simulink model "linear_equation"  (R2025b)
settings: Solver=VariableStepAuto  StartTime=0.0  StopTime=10.0  RelTol=1e-3
undefined symbols (not defined in the file or in its folder): x, x1, x2, x3
settings Model: Creator=night  LastModifiedBy=night

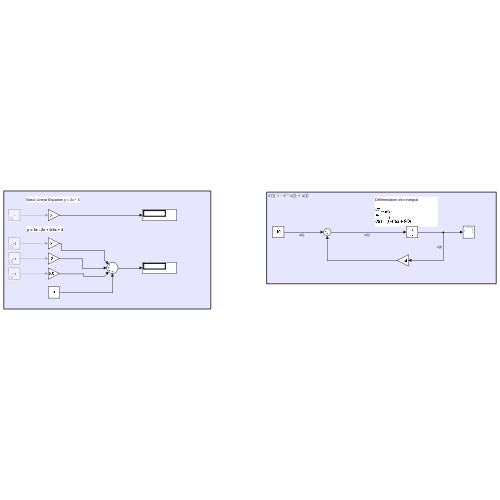
[thumbnail: Simulink's stored preview of the top-level diagram]
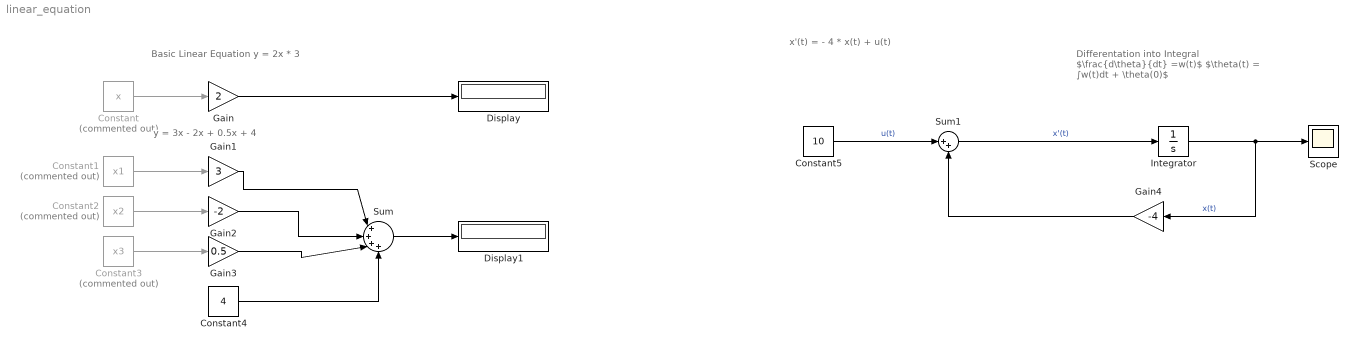
== system linear_equation ==
  note: Differentation into Integral
      |
      | $\frac{d\theta}{dt} =w(t)$
      | $\theta(t) = ∫w(t)dt + \theta(0)$
  note: x'(t) = - 4 * x(t) + u(t)
  note: y = 3x - 2x + 0.5x + 4
  note: Basic Linear Equation y = 2x * 3
  Constant : Constant  Commented=on  Value=x
  Constant1 : Constant  Commented=on  Value=x1
  Constant2 : Constant  Commented=on  Value=x2
  Constant3 : Constant  Commented=on  Value=x3
  Constant4 : Constant  Value=4
  Constant5 : Constant  Value=10
  Display : Display
  Display1 : Display
  Gain : Gain  Gain=2
  Gain1 : Gain  Gain=3
  Gain2 : Gain  Gain=-2
  Gain3 : Gain  Gain=0.5
  Gain4 : Gain  Gain=-4
  Integrator : Integrator
  Scope : Scope
      settings: ActiveDisplayYMinimum=-0.31249999999999989  ActiveDisplayYMaximum=2.8124999999999996
  Sum : Sum  Inputs=|++++
  Sum1 : Sum  Inputs=|++
  wires:
  Constant/1 -> Gain/1
  Gain/1 -> Display/1
  Gain1/1 -> Sum/1
  Constant1/1 -> Gain1/1
  Gain2/1 -> Sum/2
  Constant2/1 -> Gain2/1
  Gain3/1 -> Sum/3
  Constant3/1 -> Gain3/1
  Constant4/1 -> Sum/4
  Sum/1 -> Display1/1
  Constant5/1 -> Sum1/1  "u(t)"
  Gain4/1 -> Sum1/2
  Sum1/1 -> Integrator/1  "x'(t)"
  Integrator/1 -> Scope/1, Gain4/1  "x(t)"
